simulink model "twolevel_onephase_spwm_interleaving"  (R2015b)
settings: Solver=VariableStepAuto  StartTime=0.0  StopTime=10.0  RelTol=1e-3
libraries: powerlib x42, simulink x3, powerlib_meascontrol x1
settings Model: Creator=hakan  LastModifiedBy=hakan
settings DebuggingCC: MaxConsecutiveZCsMsg=none

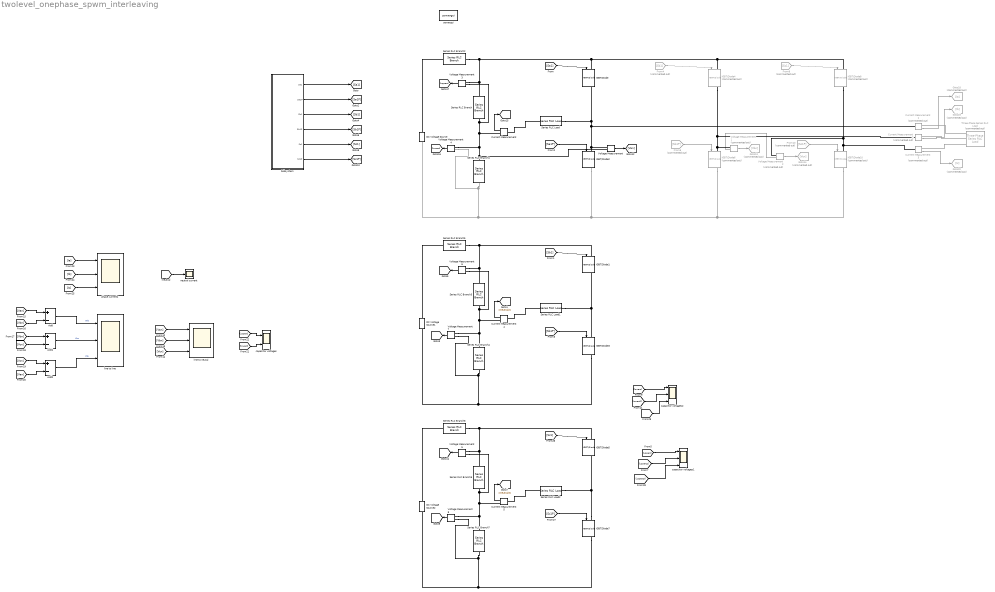
== system twolevel_onephase_spwm_interleaving ==
  Add : Sum  Inputs=+-
  Add1 : Sum  Inputs=+-
  Add2 : Sum  Inputs=+-
  Current Measurement : powerlib/Measurements/Current Measurement  PhasorSimulation=off  OutputType=Complex  PSBequivalent=0
  Current Measurement1 : powerlib/Measurements/Current Measurement  Commented=on  PhasorSimulation=off  OutputType=Complex  PSBequivalent=0
  Current Measurement2 : powerlib/Measurements/Current Measurement  Commented=on  PhasorSimulation=off  OutputType=Complex  PSBequivalent=0
  Current Measurement3 : powerlib/Measurements/Current Measurement  Commented=on  PhasorSimulation=off  OutputType=Complex  PSBequivalent=0
  Current Measurement4 : powerlib/Measurements/Current Measurement  PhasorSimulation=off  OutputType=Complex  PSBequivalent=0
  Current Measurement5 : powerlib/Measurements/Current Measurement  PhasorSimulation=off  OutputType=Complex  PSBequivalent=0
  DC Voltage Source : powerlib/Electrical Sources/DC Voltage Source  Amplitude=540  Measurements=None
  DC Voltage Source1 : powerlib/Electrical Sources/DC Voltage Source  Amplitude=540  Measurements=None
  DC Voltage Source2 : powerlib/Electrical Sources/DC Voltage Source  Amplitude=540  Measurements=None
  From10 : From  Commented=on  GotoTag=Sc1P
  From4 : From  Commented=on  GotoTag=Sb1
  From6 : From  Commented=on  GotoTag=Sb1P
  From8 : From  Commented=on  GotoTag=Sc1
  Goto13 : Goto  Commented=on  GotoTag=Vbn
  Goto14 : Goto  Commented=on  GotoTag=Vcn
  Goto18 : Goto  Commented=on  GotoTag=Ia
  Goto19 : Goto  Commented=on  GotoTag=Ib
  Goto20 : Goto  Commented=on  GotoTag=Ic
  IGBT/Diode{,1..3,5,7} (6 alike) : powerlib/Power Electronics/IGBT//Diode  Ron=1e-3  Rs=1e5  Cs=inf  Measurements=on
  IGBT/Diode{4,6,8,10} (4 alike) : powerlib/Power Electronics/IGBT//Diode  Commented=on  Ron=1e-3  Rs=1e5  Cs=inf  Measurements=on
  Series RLC Branch{,1,3..4,6..7} (6 alike) : powerlib/Elements/Series RLC Branch  LConnTagsString=__new0  RConnTagsString=__new0  BranchType=C  Resistance=1  Inductance=1e-3  SetiL0=off  InitialCurrent=0  Capacitance=1000e-6  Setx0=off  InitialVoltage=0  Measurements=None
  Series RLC Branch2 : powerlib/Elements/Series RLC Branch  LConnTagsString=__new0  RConnTagsString=__new0  BranchType=L  Resistance=1  Inductance=1e-3  SetiL0=off  InitialCurrent=0  Capacitance=1000e-6  Setx0=off  InitialVoltage=0  Measurements=None
  Series RLC Branch5 : powerlib/Elements/Series RLC Branch  LConnTagsString=__new0  RConnTagsString=__new0  BranchType=L  Resistance=1  Inductance=1e-3  SetiL0=off  InitialCurrent=0  Capacitance=1000e-6  Setx0=off  InitialVoltage=0  Measurements=None
  Series RLC Branch8 : powerlib/Elements/Series RLC Branch  LConnTagsString=__new0  RConnTagsString=__new0  BranchType=L  Resistance=1  Inductance=1e-3  SetiL0=off  InitialCurrent=0  Capacitance=1000e-6  Setx0=off  InitialVoltage=0  Measurements=None
  Series RLC Load : powerlib/Elements/Series RLC Load  LConnTagsString=a  RConnTagsString=__new0  NominalVoltage=1000  NominalFrequency=50  ActivePower=80000  InductivePower=40000  CapacitivePower=0  Setx0=off  InitialVoltage=0  SetiL0=off  InitialCurrent=0  Measurements=None  LoadType=constant Z
  Series RLC Load1 : powerlib/Elements/Series RLC Load  LConnTagsString=a  RConnTagsString=__new0  NominalVoltage=1000  NominalFrequency=50  ActivePower=80000  InductivePower=40000  CapacitivePower=0  Setx0=off  InitialVoltage=0  SetiL0=off  InitialCurrent=0  Measurements=None  LoadType=constant Z
  Series RLC Load2 : powerlib/Elements/Series RLC Load  LConnTagsString=a  RConnTagsString=__new0  NominalVoltage=1000  NominalFrequency=50  ActivePower=80000  InductivePower=40000  CapacitivePower=0  Setx0=off  InitialVoltage=0  SetiL0=off  InitialCurrent=0  Measurements=None  LoadType=constant Z
  Subsystem : Subsystem
  Three-Phase Series RLC Load : powerlib/Elements/Three-Phase Series RLC Load  Commented=on  LConnTagsString=A|B|C  Configuration=Y (grounded)  NominalVoltage=1000  Vabc=[1e3 1e3 1e3]  Vabcp=[1e3 1e3 1e3]  NominalFrequency=50  UnbalancedPower=off  ActivePower=8000  InductivePower=3870  CapacitivePower=0  Pabc=[10e3 9e3 11e3]  QLabc=[100 90 110]  QCabc=[100 90 110]  Pabcp=[10e3 9e3 11e3]  QLabcp=[100 90 110]  QCabcp=[100 90 110]  Measurements=None  LoadType=constant Z
  Voltage Measurement{,3..8} (7 alike) : powerlib/Measurements/Voltage Measurement  PhasorSimulation=off  OutputType=Complex  PSBequivalent=0
  Voltage Measurement1 : powerlib/Measurements/Voltage Measurement  Commented=on  PhasorSimulation=off  OutputType=Complex  PSBequivalent=0
  Voltage Measurement2 : powerlib/Measurements/Voltage Measurement  Commented=on  PhasorSimulation=off  OutputType=Complex  PSBequivalent=0
  capacitor voltages : Scope  NumInputPorts=2
  capacitor voltages1 : Scope  NumInputPorts=3
  capacitor voltages2 : Scope  NumInputPorts=3
  line to line : Scope  NumInputPorts=3
  line to neural : Scope  NumInputPorts=3
  neutral current : Scope
  phase currents : Scope  NumInputPorts=3
  powergui : powerlib/powergui  Priority=1  SimulationMode=Continuous  SolverType=Tustin/Backward Euler (TBE)  SampleTime=50e-6  frequency=60  SPID=off  DisableSnubberDevices=off  DisableRonSwitches=off  DisableVfSwitches=off  SwTol=0  DisplayEquations=off  Interpol=off  ExternalGateDelay=off  methode=off  Ts=10  FunctionMessages=off  echomessages=off  HookPort=off  EnableUseOfTLC=off  x0status=blocks  frequencyindice=0  Pbase=100e6  ErrMax=1e-4  Iterations=50  UnitsV=kV  UnitsW=MW  buscounter=0  RestoreLinks=warning  ResistiveCurrentMeasurement=off  Frange=[0:2:500]  Ylog=off  Xlog=on  ShowGrid=off  save=off  variable=ZData  structure=0  ZoomFFT=off  StartTime=0.0  cycles=1  DisplayStyle=1  fundamental=60  FreqAxis=off  MaxFrequency=1000  frequencyindicesteady=1  RmsSteady=1  display=off
  wires:
  Subsystem/1("Sa1 ") -> [Sa1]
  Subsystem/2(Sa1P) -> [Sa1P]
  Subsystem/3(Sb1) -> [Sb1]
  Subsystem/6(Sc1P) -> [Sc1P]
  Subsystem/5(Sc1) -> [Sc1]
  Subsystem/4(Sb1P) -> [Sb1P]
  [Sa1] -> IGBT/Diode/1
  [Sa1P] -> IGBT/Diode2/1
  From4/1 -> IGBT/Diode4/1
  From6/1 -> IGBT/Diode6/1
  From8/1 -> IGBT/Diode8/1
  From10/1 -> IGBT/Diode10/1
  Voltage Measurement/1 -> [Van]
  Voltage Measurement1/1 -> Goto13/1
  Voltage Measurement2/1 -> Goto14/1
  Voltage Measurement3/1 -> [upperc]
  Voltage Measurement4/1 -> [lowerc]
  Current Measurement/1 -> [Ineutral]
  [Ineutral] -> neutral current/1
  Current Measurement1/1 -> Goto18/1
  Current Measurement2/1 -> Goto19/1
  Current Measurement3/1 -> Goto20/1
  [Ib] -> phase currents/2
  [Ia] -> phase currents/1
  [Ic] -> phase currents/3
  [Van] -> Add/1
  [Vbn] -> Add/2
  Add/1 -> line to line/1  "Vab"
  [Vbn] -> Add1/1
  [Vcn] -> Add1/2
  Add1/1 -> line to line/2  "Vbc"
  [Vcn] -> Add2/1
  [Van] -> Add2/2
  Add2/1 -> line to line/3  "Vca"
  [Van] -> line to neural/1
  [Vbn] -> line to neural/2
  [Vcn] -> line to neural/3
  [lowerc] -> capacitor voltages/2
  [upperc] -> capacitor voltages/1
  [Sb1] -> IGBT/Diode1/1
  [Sb1P] -> IGBT/Diode3/1
  Voltage Measurement6/1 -> [upperc2]
  Voltage Measurement7/1 -> [lowerc2]
  Current Measurement4/1 -> [Ineutral2]
  [upperc] -> capacitor voltages1/1
  [upperc2] -> capacitor voltages1/2
  [lowerc] -> capacitor voltages2/1
  [lowerc2] -> capacitor voltages2/2
  [Sc1] -> IGBT/Diode5/1
  [Sc1P] -> IGBT/Diode7/1
  Voltage Measurement5/1 -> [upperc3]
  Voltage Measurement8/1 -> [lowerc3]
  Current Measurement5/1 -> [Ineutral3]
  [upperc3] -> capacitor voltages1/3
  [lowerc3] -> capacitor voltages2/3
  connections:
  Voltage Measurement3/LConn1 -- IGBT/Diode/LConn1 -- IGBT/Diode4/LConn1 -- IGBT/Diode8/LConn1 -- Series RLC Branch2/LConn1 -- Series RLC Branch/LConn1
  IGBT/Diode7/RConn1 -- Series RLC Branch7/RConn1 -- Voltage Measurement8/LConn2 -- DC Voltage Source2/LConn1
  IGBT/Diode2/LConn1 -- Voltage Measurement/LConn1 -- Current Measurement1/LConn1 -- Series RLC Load/RConn1 -- IGBT/Diode/RConn1
  Voltage Measurement1/LConn2 -- Voltage Measurement2/LConn2
  IGBT/Diode6/LConn1 -- Voltage Measurement1/LConn1 -- IGBT/Diode4/RConn1 -- Current Measurement2/LConn1
  IGBT/Diode8/RConn1 -- Voltage Measurement2/LConn1 -- Current Measurement3/LConn1 -- IGBT/Diode10/LConn1
  Series RLC Branch1/LConn1 -- Current Measurement/RConn1 -- Series RLC Branch/RConn1 -- Voltage Measurement3/LConn2 -- Voltage Measurement4/LConn1 -- Voltage Measurement/LConn2
  Three-Phase Series RLC Load/LConn1 -- Current Measurement1/RConn1
  Three-Phase Series RLC Load/LConn3 -- Current Measurement3/RConn1
  Three-Phase Series RLC Load/LConn2 -- Current Measurement2/RConn1
  DC Voltage Source/RConn1 -- Series RLC Branch2/RConn1
  Series RLC Load/LConn1 -- Current Measurement/LConn1
  Series RLC Load1/RConn1 -- IGBT/Diode3/LConn1 -- IGBT/Diode1/RConn1
  DC Voltage Source1/RConn1 -- Series RLC Branch5/RConn1
  Series RLC Load1/LConn1 -- Current Measurement4/LConn1
  IGBT/Diode7/LConn1 -- Series RLC Load2/RConn1 -- IGBT/Diode5/RConn1
  Series RLC Load2/LConn1 -- Current Measurement5/LConn1
  DC Voltage Source2/RConn1 -- Series RLC Branch8/RConn1
  IGBT/Diode6/RConn1 -- IGBT/Diode10/RConn1 -- IGBT/Diode2/RConn1 -- Series RLC Branch1/RConn1 -- Voltage Measurement4/LConn2 -- DC Voltage Source/LConn1
  Series RLC Branch5/LConn1 -- IGBT/Diode1/LConn1 -- Voltage Measurement6/LConn1 -- Series RLC Branch3/LConn1
  Current Measurement5/RConn1 -- Series RLC Branch7/LConn1 -- Voltage Measurement8/LConn1 -- Series RLC Branch6/RConn1 -- Voltage Measurement5/LConn2
  Series RLC Branch8/LConn1 -- IGBT/Diode5/LConn1 -- Series RLC Branch6/LConn1 -- Voltage Measurement5/LConn1
  Voltage Measurement7/LConn2 -- Series RLC Branch4/RConn1 -- IGBT/Diode3/RConn1 -- DC Voltage Source1/LConn1
  Voltage Measurement6/LConn2 -- Series RLC Branch3/RConn1 -- Current Measurement4/RConn1 -- Voltage Measurement7/LConn1 -- Series RLC Branch4/LConn1

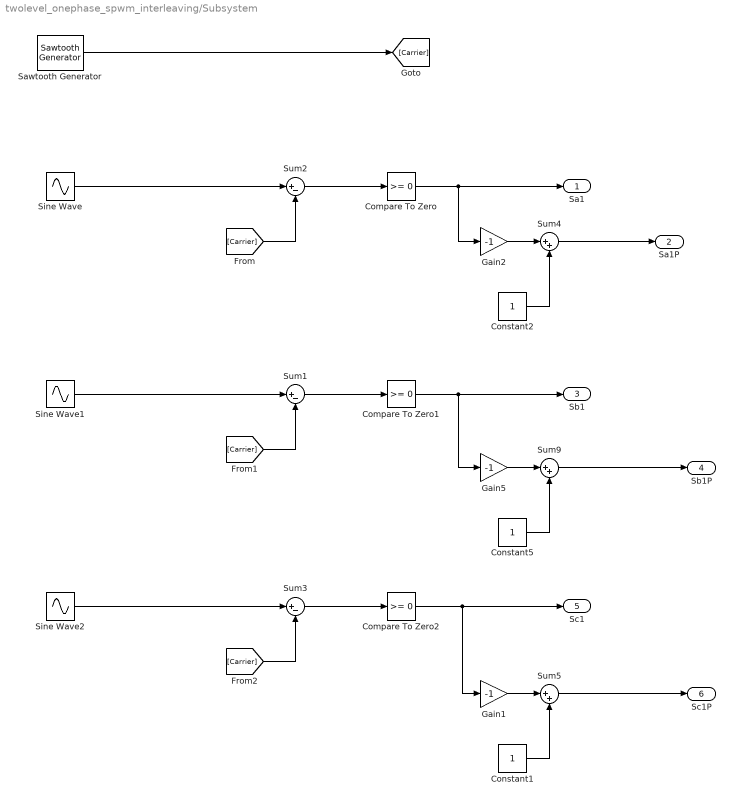
== system twolevel_onephase_spwm_interleaving/Subsystem ==
  Compare To Zero : simulink/Logic and Bit Operations/Compare To Zero  relop=>=  OutDataTypeStr=boolean
  Compare To Zero1 : simulink/Logic and Bit Operations/Compare To Zero  relop=>=  OutDataTypeStr=boolean
  Compare To Zero2 : simulink/Logic and Bit Operations/Compare To Zero  relop=>=  OutDataTypeStr=boolean
  Constant1 : Constant
  Constant2 : Constant
  Constant5 : Constant
  Gain1 : Gain  Gain=-1
  Gain2 : Gain  Gain=-1
  Gain5 : Gain  Gain=-1
  Sawtooth Generator : powerlib_meascontrol/Pulse & Signal Generators/Sawtooth Generator  Freq=2e3  Phase=180  Ts=0
  Sine Wave : Sin  Amplitude=0.8  Frequency=100*pi  SampleTime=0
  Sine Wave1 : Sin  Amplitude=0.8  Frequency=100*pi  Phase=2*pi/3  SampleTime=0
  Sine Wave2 : Sin  Amplitude=0.8  Frequency=100*pi  Phase=4*pi/3  SampleTime=0
  Sum1 : Sum  Inputs=|+-
  Sum2 : Sum  Inputs=|+-
  Sum3 : Sum  Inputs=|+-
  Sum4 : Sum  Inputs=|++
  Sum5 : Sum  Inputs=|++
  Sum9 : Sum  Inputs=|++
  "Sa1 " : Outport
  Sa1P : Outport  Port=2
  Sb1 : Outport  Port=3
  Sb1P : Outport  Port=4
  Sc1 : Outport  Port=5
  Sc1P : Outport  Port=6
  wires:
  Sine Wave/1 -> Sum2/1
  Sum4/1 -> Sa1P/1
  Gain2/1 -> Sum4/1
  Constant2/1 -> Sum4/2
  Compare To Zero/1 -> "Sa1 "/1, Gain2/1
  Sum2/1 -> Compare To Zero/1
  [Carrier] -> Sum2/2
  Sawtooth Generator/1 -> [Carrier]
  Compare To Zero1/1 -> Gain5/1, Sb1/1
  Sine Wave1/1 -> Sum1/1
  [Carrier] -> Sum1/2
  Compare To Zero2/1 -> Gain1/1, Sc1/1
  Sine Wave2/1 -> Sum3/1
  [Carrier] -> Sum3/2
  Sum1/1 -> Compare To Zero1/1
  Gain5/1 -> Sum9/1
  Sum9/1 -> Sb1P/1
  Constant5/1 -> Sum9/2
  Constant1/1 -> Sum5/2
  Sum5/1 -> Sc1P/1
  Sum3/1 -> Compare To Zero2/1
  Gain1/1 -> Sum5/1
